simulink model "TST_EnvT_VD"  (R2016b)
settings: Solver=FixedStepDiscrete  StartTime=0.0  StopTime=simTime  FixedStep=sampleTime  RelTol=1e-3
values from neighbouring files (symbols this model uses):
  testCase = 1    [initTST_EnvT_VD_001.m]    (also in initTST_EnvT_VD_002.m = 2; initTST_EnvT_VD_003.m = 3; initTST_EnvT_VD_004.m = 4)
libraries: simulink x9, UnitTest_Lib x4
settings Model: Creator=liangyunbo  LastModifiedBy=liangyunbo
settings DebuggingCC: SignalRangeChecking=error

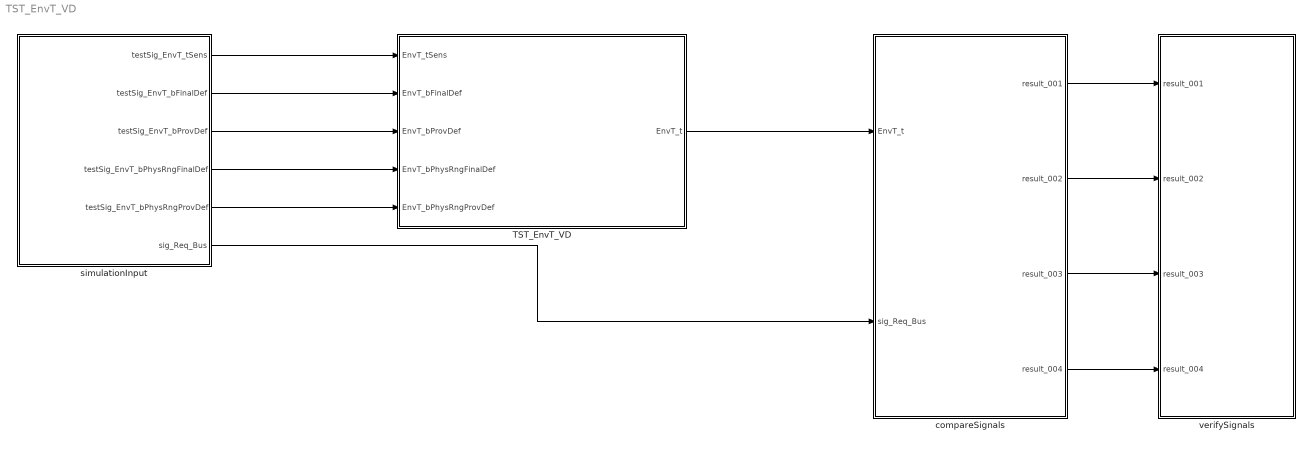
== system TST_EnvT_VD ==
  TST_EnvT_VD : Subsystem
  compareSignals : Subsystem
  simulationInput : Subsystem
  verifySignals : Subsystem
  wires:
  simulationInput/1(testSig_EnvT_tSens) -> TST_EnvT_VD/1(EnvT_tSens)
  simulationInput/2(testSig_EnvT_bFinalDef) -> TST_EnvT_VD/2(EnvT_bFinalDef)
  simulationInput/3(testSig_EnvT_bProvDef) -> TST_EnvT_VD/3(EnvT_bProvDef)
  simulationInput/4(testSig_EnvT_bPhysRngFinalDef) -> TST_EnvT_VD/4(EnvT_bPhysRngFinalDef)
  simulationInput/5(testSig_EnvT_bPhysRngProvDef) -> TST_EnvT_VD/5(EnvT_bPhysRngProvDef)
  TST_EnvT_VD/1(EnvT_t) -> compareSignals/1(EnvT_t)
  simulationInput/6(sig_Req_Bus) -> compareSignals/2(sig_Req_Bus)
  compareSignals/1(result_001) -> verifySignals/1(result_001)
  compareSignals/2(result_002) -> verifySignals/2(result_002)
  compareSignals/3(result_003) -> verifySignals/3(result_003)
  compareSignals/4(result_004) -> verifySignals/4(result_004)

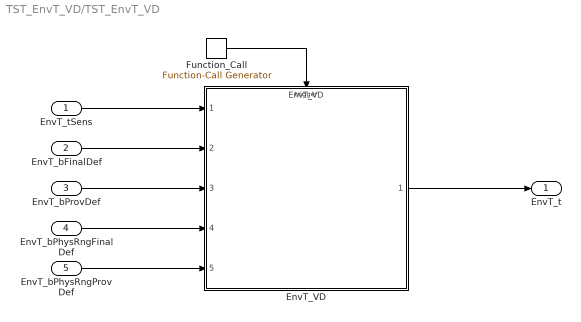
== system TST_EnvT_VD/TST_EnvT_VD ==
  EnvT_tSens : Inport
  EnvT_bFinalDef : Inport  Port=2
  EnvT_bProvDef : Inport  Port=3
  EnvT_bPhysRngFinalDef : Inport  Port=4
  EnvT_bPhysRngProvDef : Inport  Port=5
  EnvT_VD : ModelReference  ModelNameDialog=EnvT_VD  SimulationMode=Normal  ModelReferenceVersion=1.9  TriggerPortName=function  TriggerPortTriggerType=function-call  TriggerPortStatesWhenEnabling=held
  Function_Call : simulink/Ports & Subsystems/Function-Call Generator  sample_time=sampleTime  numberOfIterations=1
  EnvT_t : Outport
  wires:
  Function_Call/1 -> EnvT_VD/Trigger
  EnvT_tSens/1 -> EnvT_VD/1
  EnvT_bFinalDef/1 -> EnvT_VD/2
  EnvT_bProvDef/1 -> EnvT_VD/3
  EnvT_bPhysRngFinalDef/1 -> EnvT_VD/4
  EnvT_bPhysRngProvDef/1 -> EnvT_VD/5
  EnvT_VD/1 -> EnvT_t/1

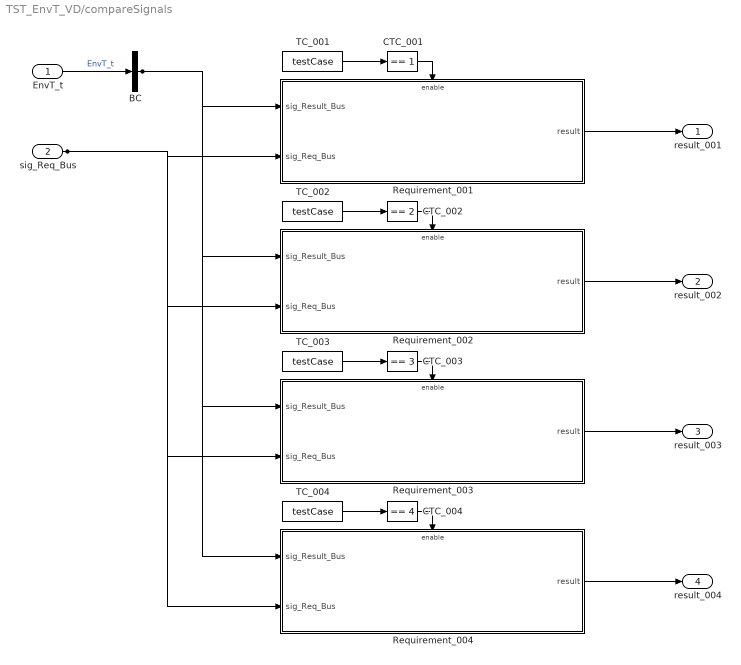
== system TST_EnvT_VD/compareSignals ==
  EnvT_t : Inport
  sig_Req_Bus : Inport  Port=2
  BC : BusCreator  Inputs=1
  CTC_001 : simulink/Logic and Bit Operations/Compare To Constant  relop===  const=1  OutDataTypeStr=boolean
  CTC_002 : simulink/Logic and Bit Operations/Compare To Constant  relop===  const=2  OutDataTypeStr=boolean
  CTC_003 : simulink/Logic and Bit Operations/Compare To Constant  relop===  const=3  OutDataTypeStr=boolean
  CTC_004 : simulink/Logic and Bit Operations/Compare To Constant  relop===  const=4  OutDataTypeStr=boolean
  Requirement_001 : Subsystem
  Requirement_002 : Subsystem
  Requirement_003 : Subsystem
  Requirement_004 : Subsystem
  TC_001 : Constant  Value=testCase
  TC_002 : Constant  Value=testCase
  TC_003 : Constant  Value=testCase
  TC_004 : Constant  Value=testCase
  result_001 : Outport
  result_002 : Outport  Port=2
  result_003 : Outport  Port=3
  result_004 : Outport  Port=4
  wires:
  EnvT_t/1 -> BC/1  "EnvT_t"
  TC_001/1 -> CTC_001/1
  CTC_001/1 -> Requirement_001/Enable
  sig_Req_Bus/1 -> Requirement_001/2(sig_Req_Bus), Requirement_002/2(sig_Req_Bus), Requirement_003/2(sig_Req_Bus), Requirement_004/2(sig_Req_Bus)
  BC/1 -> Requirement_001/1(sig_Result_Bus), Requirement_002/1(sig_Result_Bus), Requirement_003/1(sig_Result_Bus), Requirement_004/1(sig_Result_Bus)
  Requirement_001/1(result) -> result_001/1
  TC_002/1 -> CTC_002/1
  CTC_002/1 -> Requirement_002/Enable
  Requirement_002/1(result) -> result_002/1
  TC_003/1 -> CTC_003/1
  CTC_003/1 -> Requirement_003/Enable
  Requirement_003/1(result) -> result_003/1
  TC_004/1 -> CTC_004/1
  CTC_004/1 -> Requirement_004/Enable
  Requirement_004/1(result) -> result_004/1

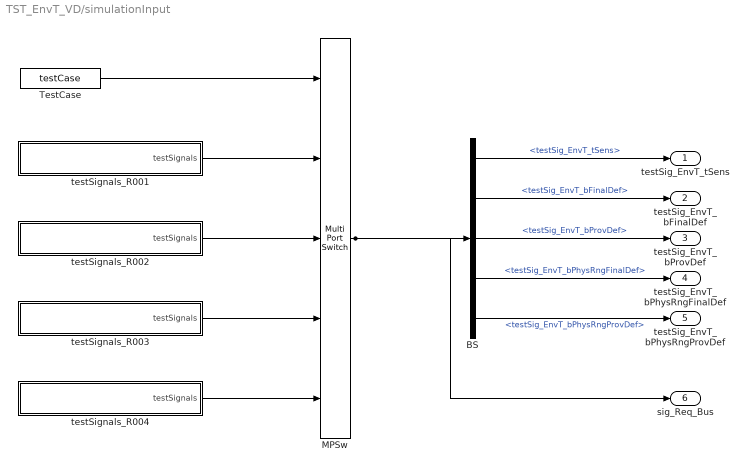
== system TST_EnvT_VD/simulationInput ==
  BS : BusSelector  OutputSignals=testSig_EnvT_tSens,testSig_EnvT_bFinalDef,testSig_EnvT_bProvDef,testSig_EnvT_bPhysRngFinalDef,testSig_EnvT_bPhysRngProvDef
  MPSw : MultiPortSwitch  Inputs=4  SaturateOnIntegerOverflow=on  InputSameDT=on
  TestCase : Constant  Value=testCase
  testSignals_R001 : Subsystem
  testSignals_R002 : Subsystem
  testSignals_R003 : Subsystem
  testSignals_R004 : Subsystem
  testSig_EnvT_tSens : Outport
  testSig_EnvT_bFinalDef : Outport  Port=2
  testSig_EnvT_bProvDef : Outport  Port=3
  testSig_EnvT_bPhysRngFinalDef : Outport  Port=4
  testSig_EnvT_bPhysRngProvDef : Outport  Port=5
  sig_Req_Bus : Outport  Port=6
  wires:
  BS/1 -> testSig_EnvT_tSens/1  "<testSig_EnvT_tSens>"
  BS/2 -> testSig_EnvT_bFinalDef/1  "<testSig_EnvT_bFinalDef>"
  BS/3 -> testSig_EnvT_bProvDef/1  "<testSig_EnvT_bProvDef>"
  BS/4 -> testSig_EnvT_bPhysRngFinalDef/1  "<testSig_EnvT_bPhysRngFinalDef>"
  BS/5 -> testSig_EnvT_bPhysRngProvDef/1  "<testSig_EnvT_bPhysRngProvDef>"
  MPSw/1 -> BS/1, sig_Req_Bus/1
  TestCase/1 -> MPSw/1
  testSignals_R001/1(testSignals) -> MPSw/2
  testSignals_R002/1(testSignals) -> MPSw/3
  testSignals_R003/1(testSignals) -> MPSw/4
  testSignals_R004/1(testSignals) -> MPSw/5

== system TST_EnvT_VD/verifySignals ==
  result_001 : Inport
  result_002 : Inport  Port=2
  result_003 : Inport  Port=3
  result_004 : Inport  Port=4
  Assertion_001 : Assertion  Enabled=off
  Assertion_002 : Assertion  Enabled=off
  Assertion_003 : Assertion  Enabled=off
  Assertion_004 : Assertion  Enabled=off
  wires:
  result_001/1 -> Assertion_001/1
  result_002/1 -> Assertion_002/1
  result_003/1 -> Assertion_003/1
  result_004/1 -> Assertion_004/1

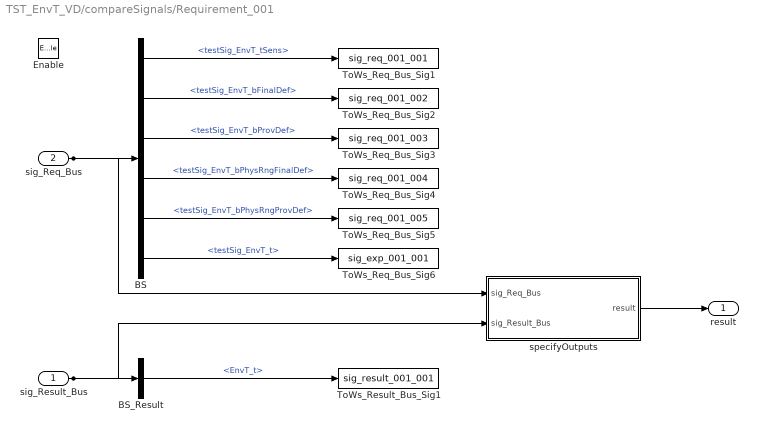
== system TST_EnvT_VD/compareSignals/Requirement_001 ==
  sig_Result_Bus : Inport
  sig_Req_Bus : Inport  Port=2
  Enable : EnablePort
  BS : BusSelector  OutputSignals=testSig_EnvT_tSens,testSig_EnvT_bFinalDef,testSig_EnvT_bProvDef,testSig_EnvT_bPhysRngFinalDef,testSig_EnvT_bPhysRngProvDef,testSig_EnvT_t
  BS_Result : BusSelector  OutputSignals=EnvT_t
  ToWs_Req_Bus_Sig1 : ToWorkspace  VariableName=sig_req_001_001  SaveFormat=Structure With Time
  ToWs_Req_Bus_Sig2 : ToWorkspace  VariableName=sig_req_001_002  SaveFormat=Structure With Time
  ToWs_Req_Bus_Sig3 : ToWorkspace  VariableName=sig_req_001_003  SaveFormat=Structure With Time
  ToWs_Req_Bus_Sig4 : ToWorkspace  VariableName=sig_req_001_004  SaveFormat=Structure With Time
  ToWs_Req_Bus_Sig5 : ToWorkspace  VariableName=sig_req_001_005  SaveFormat=Structure With Time
  ToWs_Req_Bus_Sig6 : ToWorkspace  VariableName=sig_exp_001_001  SaveFormat=Structure With Time
  ToWs_Result_Bus_Sig1 : ToWorkspace  VariableName=sig_result_001_001  SaveFormat=Structure With Time
  specifyOutputs : Subsystem
  result : Outport
  wires:
  sig_Req_Bus/1 -> BS/1, specifyOutputs/1(sig_Req_Bus)
  BS/1 -> ToWs_Req_Bus_Sig1/1  "<testSig_EnvT_tSens>"
  BS/2 -> ToWs_Req_Bus_Sig2/1  "<testSig_EnvT_bFinalDef>"
  BS/3 -> ToWs_Req_Bus_Sig3/1  "<testSig_EnvT_bProvDef>"
  BS/4 -> ToWs_Req_Bus_Sig4/1  "<testSig_EnvT_bPhysRngFinalDef>"
  BS/5 -> ToWs_Req_Bus_Sig5/1  "<testSig_EnvT_bPhysRngProvDef>"
  BS/6 -> ToWs_Req_Bus_Sig6/1  "<testSig_EnvT_t>"
  sig_Result_Bus/1 -> BS_Result/1, specifyOutputs/2(sig_Result_Bus)
  BS_Result/1 -> ToWs_Result_Bus_Sig1/1  "<EnvT_t>"
  specifyOutputs/1(result) -> result/1

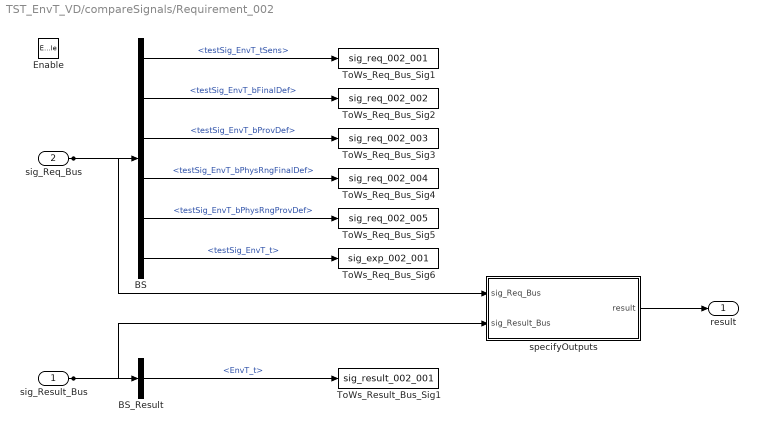
== system TST_EnvT_VD/compareSignals/Requirement_002 ==
  sig_Result_Bus : Inport
  sig_Req_Bus : Inport  Port=2
  Enable : EnablePort
  BS : BusSelector  OutputSignals=testSig_EnvT_tSens,testSig_EnvT_bFinalDef,testSig_EnvT_bProvDef,testSig_EnvT_bPhysRngFinalDef,testSig_EnvT_bPhysRngProvDef,testSig_EnvT_t
  BS_Result : BusSelector  OutputSignals=EnvT_t
  ToWs_Req_Bus_Sig1 : ToWorkspace  VariableName=sig_req_002_001  SaveFormat=Structure With Time
  ToWs_Req_Bus_Sig2 : ToWorkspace  VariableName=sig_req_002_002  SaveFormat=Structure With Time
  ToWs_Req_Bus_Sig3 : ToWorkspace  VariableName=sig_req_002_003  SaveFormat=Structure With Time
  ToWs_Req_Bus_Sig4 : ToWorkspace  VariableName=sig_req_002_004  SaveFormat=Structure With Time
  ToWs_Req_Bus_Sig5 : ToWorkspace  VariableName=sig_req_002_005  SaveFormat=Structure With Time
  ToWs_Req_Bus_Sig6 : ToWorkspace  VariableName=sig_exp_002_001  SaveFormat=Structure With Time
  ToWs_Result_Bus_Sig1 : ToWorkspace  VariableName=sig_result_002_001  SaveFormat=Structure With Time
  specifyOutputs : Subsystem
  result : Outport
  wires:
  sig_Req_Bus/1 -> BS/1, specifyOutputs/1(sig_Req_Bus)
  BS/1 -> ToWs_Req_Bus_Sig1/1  "<testSig_EnvT_tSens>"
  BS/2 -> ToWs_Req_Bus_Sig2/1  "<testSig_EnvT_bFinalDef>"
  BS/3 -> ToWs_Req_Bus_Sig3/1  "<testSig_EnvT_bProvDef>"
  BS/4 -> ToWs_Req_Bus_Sig4/1  "<testSig_EnvT_bPhysRngFinalDef>"
  BS/5 -> ToWs_Req_Bus_Sig5/1  "<testSig_EnvT_bPhysRngProvDef>"
  BS/6 -> ToWs_Req_Bus_Sig6/1  "<testSig_EnvT_t>"
  sig_Result_Bus/1 -> BS_Result/1, specifyOutputs/2(sig_Result_Bus)
  BS_Result/1 -> ToWs_Result_Bus_Sig1/1  "<EnvT_t>"
  specifyOutputs/1(result) -> result/1

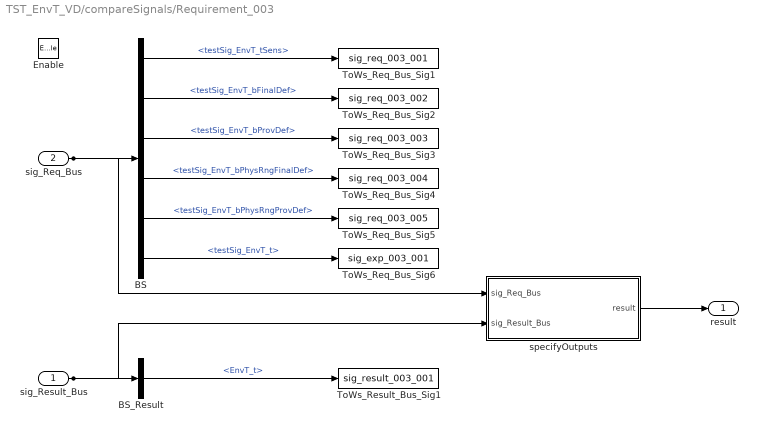
== system TST_EnvT_VD/compareSignals/Requirement_003 ==
  sig_Result_Bus : Inport
  sig_Req_Bus : Inport  Port=2
  Enable : EnablePort
  BS : BusSelector  OutputSignals=testSig_EnvT_tSens,testSig_EnvT_bFinalDef,testSig_EnvT_bProvDef,testSig_EnvT_bPhysRngFinalDef,testSig_EnvT_bPhysRngProvDef,testSig_EnvT_t
  BS_Result : BusSelector  OutputSignals=EnvT_t
  ToWs_Req_Bus_Sig1 : ToWorkspace  VariableName=sig_req_003_001  SaveFormat=Structure With Time
  ToWs_Req_Bus_Sig2 : ToWorkspace  VariableName=sig_req_003_002  SaveFormat=Structure With Time
  ToWs_Req_Bus_Sig3 : ToWorkspace  VariableName=sig_req_003_003  SaveFormat=Structure With Time
  ToWs_Req_Bus_Sig4 : ToWorkspace  VariableName=sig_req_003_004  SaveFormat=Structure With Time
  ToWs_Req_Bus_Sig5 : ToWorkspace  VariableName=sig_req_003_005  SaveFormat=Structure With Time
  ToWs_Req_Bus_Sig6 : ToWorkspace  VariableName=sig_exp_003_001  SaveFormat=Structure With Time
  ToWs_Result_Bus_Sig1 : ToWorkspace  VariableName=sig_result_003_001  SaveFormat=Structure With Time
  specifyOutputs : Subsystem
  result : Outport
  wires:
  sig_Req_Bus/1 -> BS/1, specifyOutputs/1(sig_Req_Bus)
  BS/1 -> ToWs_Req_Bus_Sig1/1  "<testSig_EnvT_tSens>"
  BS/2 -> ToWs_Req_Bus_Sig2/1  "<testSig_EnvT_bFinalDef>"
  BS/3 -> ToWs_Req_Bus_Sig3/1  "<testSig_EnvT_bProvDef>"
  BS/4 -> ToWs_Req_Bus_Sig4/1  "<testSig_EnvT_bPhysRngFinalDef>"
  BS/5 -> ToWs_Req_Bus_Sig5/1  "<testSig_EnvT_bPhysRngProvDef>"
  BS/6 -> ToWs_Req_Bus_Sig6/1  "<testSig_EnvT_t>"
  sig_Result_Bus/1 -> BS_Result/1, specifyOutputs/2(sig_Result_Bus)
  BS_Result/1 -> ToWs_Result_Bus_Sig1/1  "<EnvT_t>"
  specifyOutputs/1(result) -> result/1

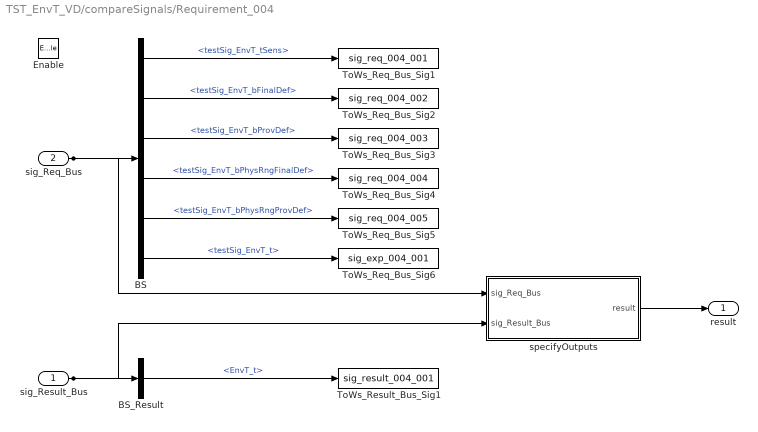
== system TST_EnvT_VD/compareSignals/Requirement_004 ==
  sig_Result_Bus : Inport
  sig_Req_Bus : Inport  Port=2
  Enable : EnablePort
  BS : BusSelector  OutputSignals=testSig_EnvT_tSens,testSig_EnvT_bFinalDef,testSig_EnvT_bProvDef,testSig_EnvT_bPhysRngFinalDef,testSig_EnvT_bPhysRngProvDef,testSig_EnvT_t
  BS_Result : BusSelector  OutputSignals=EnvT_t
  ToWs_Req_Bus_Sig1 : ToWorkspace  VariableName=sig_req_004_001  SaveFormat=Structure With Time
  ToWs_Req_Bus_Sig2 : ToWorkspace  VariableName=sig_req_004_002  SaveFormat=Structure With Time
  ToWs_Req_Bus_Sig3 : ToWorkspace  VariableName=sig_req_004_003  SaveFormat=Structure With Time
  ToWs_Req_Bus_Sig4 : ToWorkspace  VariableName=sig_req_004_004  SaveFormat=Structure With Time
  ToWs_Req_Bus_Sig5 : ToWorkspace  VariableName=sig_req_004_005  SaveFormat=Structure With Time
  ToWs_Req_Bus_Sig6 : ToWorkspace  VariableName=sig_exp_004_001  SaveFormat=Structure With Time
  ToWs_Result_Bus_Sig1 : ToWorkspace  VariableName=sig_result_004_001  SaveFormat=Structure With Time
  specifyOutputs : Subsystem
  result : Outport
  wires:
  sig_Req_Bus/1 -> BS/1, specifyOutputs/1(sig_Req_Bus)
  BS/1 -> ToWs_Req_Bus_Sig1/1  "<testSig_EnvT_tSens>"
  BS/2 -> ToWs_Req_Bus_Sig2/1  "<testSig_EnvT_bFinalDef>"
  BS/3 -> ToWs_Req_Bus_Sig3/1  "<testSig_EnvT_bProvDef>"
  BS/4 -> ToWs_Req_Bus_Sig4/1  "<testSig_EnvT_bPhysRngFinalDef>"
  BS/5 -> ToWs_Req_Bus_Sig5/1  "<testSig_EnvT_bPhysRngProvDef>"
  BS/6 -> ToWs_Req_Bus_Sig6/1  "<testSig_EnvT_t>"
  sig_Result_Bus/1 -> BS_Result/1, specifyOutputs/2(sig_Result_Bus)
  BS_Result/1 -> ToWs_Result_Bus_Sig1/1  "<EnvT_t>"
  specifyOutputs/1(result) -> result/1

== system TST_EnvT_VD/simulationInput/testSignals_R001 ==
  BC : BusCreator  Inputs=6
  spec_EnvT_bFinalDef : FromWorkspace  VariableName=testSig_EnvT_bFinalDef  Interpolate=off  OutputAfterFinalValue=Holding final value
  spec_EnvT_bPhysRngFinalDef : FromWorkspace  VariableName=testSig_EnvT_bPhysRngFinalDef  Interpolate=off  OutputAfterFinalValue=Holding final value
  spec_EnvT_bPhysRngProvDef : FromWorkspace  VariableName=testSig_EnvT_bPhysRngProvDef  Interpolate=off  OutputAfterFinalValue=Holding final value
  spec_EnvT_bProvDef : FromWorkspace  VariableName=testSig_EnvT_bProvDef  Interpolate=off  OutputAfterFinalValue=Holding final value
  spec_EnvT_t : FromWorkspace  VariableName=testSig_EnvT_t  Interpolate=off  OutputAfterFinalValue=Holding final value
  spec_EnvT_tSens : FromWorkspace  VariableName=testSig_EnvT_tSens  Interpolate=off  OutputAfterFinalValue=Holding final value
  testSignals : Outport
  wires:
  BC/1 -> testSignals/1
  spec_EnvT_tSens/1 -> BC/1  "testSig_EnvT_tSens"
  spec_EnvT_bFinalDef/1 -> BC/2  "testSig_EnvT_bFinalDef"
  spec_EnvT_bProvDef/1 -> BC/3  "testSig_EnvT_bProvDef"
  spec_EnvT_bPhysRngFinalDef/1 -> BC/4  "testSig_EnvT_bPhysRngFinalDef"
  spec_EnvT_bPhysRngProvDef/1 -> BC/5  "testSig_EnvT_bPhysRngProvDef"
  spec_EnvT_t/1 -> BC/6  "testSig_EnvT_t"

== system TST_EnvT_VD/simulationInput/testSignals_R002 ==
  BC : BusCreator  Inputs=6
  spec_EnvT_bFinalDef : FromWorkspace  VariableName=testSig_EnvT_bFinalDef  Interpolate=off  OutputAfterFinalValue=Holding final value
  spec_EnvT_bPhysRngFinalDef : FromWorkspace  VariableName=testSig_EnvT_bPhysRngFinalDef  Interpolate=off  OutputAfterFinalValue=Holding final value
  spec_EnvT_bPhysRngProvDef : FromWorkspace  VariableName=testSig_EnvT_bPhysRngProvDef  Interpolate=off  OutputAfterFinalValue=Holding final value
  spec_EnvT_bProvDef : FromWorkspace  VariableName=testSig_EnvT_bProvDef  Interpolate=off  OutputAfterFinalValue=Holding final value
  spec_EnvT_t : FromWorkspace  VariableName=testSig_EnvT_t  Interpolate=off  OutputAfterFinalValue=Holding final value
  spec_EnvT_tSens : FromWorkspace  VariableName=testSig_EnvT_tSens  Interpolate=off  OutputAfterFinalValue=Holding final value
  testSignals : Outport
  wires:
  BC/1 -> testSignals/1
  spec_EnvT_tSens/1 -> BC/1  "testSig_EnvT_tSens"
  spec_EnvT_bFinalDef/1 -> BC/2  "testSig_EnvT_bFinalDef"
  spec_EnvT_bProvDef/1 -> BC/3  "testSig_EnvT_bProvDef"
  spec_EnvT_bPhysRngFinalDef/1 -> BC/4  "testSig_EnvT_bPhysRngFinalDef"
  spec_EnvT_bPhysRngProvDef/1 -> BC/5  "testSig_EnvT_bPhysRngProvDef"
  spec_EnvT_t/1 -> BC/6  "testSig_EnvT_t"

== system TST_EnvT_VD/simulationInput/testSignals_R003 ==
  BC : BusCreator  Inputs=6
  spec_EnvT_bFinalDef : FromWorkspace  VariableName=testSig_EnvT_bFinalDef  Interpolate=off  OutputAfterFinalValue=Holding final value
  spec_EnvT_bPhysRngFinalDef : FromWorkspace  VariableName=testSig_EnvT_bPhysRngFinalDef  Interpolate=off  OutputAfterFinalValue=Holding final value
  spec_EnvT_bPhysRngProvDef : FromWorkspace  VariableName=testSig_EnvT_bPhysRngProvDef  Interpolate=off  OutputAfterFinalValue=Holding final value
  spec_EnvT_bProvDef : FromWorkspace  VariableName=testSig_EnvT_bProvDef  Interpolate=off  OutputAfterFinalValue=Holding final value
  spec_EnvT_t : FromWorkspace  VariableName=testSig_EnvT_t  Interpolate=off  OutputAfterFinalValue=Holding final value
  spec_EnvT_tSens : FromWorkspace  VariableName=testSig_EnvT_tSens  Interpolate=off  OutputAfterFinalValue=Holding final value
  testSignals : Outport
  wires:
  BC/1 -> testSignals/1
  spec_EnvT_tSens/1 -> BC/1  "testSig_EnvT_tSens"
  spec_EnvT_bFinalDef/1 -> BC/2  "testSig_EnvT_bFinalDef"
  spec_EnvT_bProvDef/1 -> BC/3  "testSig_EnvT_bProvDef"
  spec_EnvT_bPhysRngFinalDef/1 -> BC/4  "testSig_EnvT_bPhysRngFinalDef"
  spec_EnvT_bPhysRngProvDef/1 -> BC/5  "testSig_EnvT_bPhysRngProvDef"
  spec_EnvT_t/1 -> BC/6  "testSig_EnvT_t"

== system TST_EnvT_VD/simulationInput/testSignals_R004 ==
  BC : BusCreator  Inputs=6
  spec_EnvT_bFinalDef : FromWorkspace  VariableName=testSig_EnvT_bFinalDef  Interpolate=off  OutputAfterFinalValue=Holding final value
  spec_EnvT_bPhysRngFinalDef : FromWorkspace  VariableName=testSig_EnvT_bPhysRngFinalDef  Interpolate=off  OutputAfterFinalValue=Holding final value
  spec_EnvT_bPhysRngProvDef : FromWorkspace  VariableName=testSig_EnvT_bPhysRngProvDef  Interpolate=off  OutputAfterFinalValue=Holding final value
  spec_EnvT_bProvDef : FromWorkspace  VariableName=testSig_EnvT_bProvDef  Interpolate=off  OutputAfterFinalValue=Holding final value
  spec_EnvT_t : FromWorkspace  VariableName=testSig_EnvT_t  Interpolate=off  OutputAfterFinalValue=Holding final value
  spec_EnvT_tSens : FromWorkspace  VariableName=testSig_EnvT_tSens  Interpolate=off  OutputAfterFinalValue=Holding final value
  testSignals : Outport
  wires:
  BC/1 -> testSignals/1
  spec_EnvT_tSens/1 -> BC/1  "testSig_EnvT_tSens"
  spec_EnvT_bFinalDef/1 -> BC/2  "testSig_EnvT_bFinalDef"
  spec_EnvT_bProvDef/1 -> BC/3  "testSig_EnvT_bProvDef"
  spec_EnvT_bPhysRngFinalDef/1 -> BC/4  "testSig_EnvT_bPhysRngFinalDef"
  spec_EnvT_bPhysRngProvDef/1 -> BC/5  "testSig_EnvT_bPhysRngProvDef"
  spec_EnvT_t/1 -> BC/6  "testSig_EnvT_t"

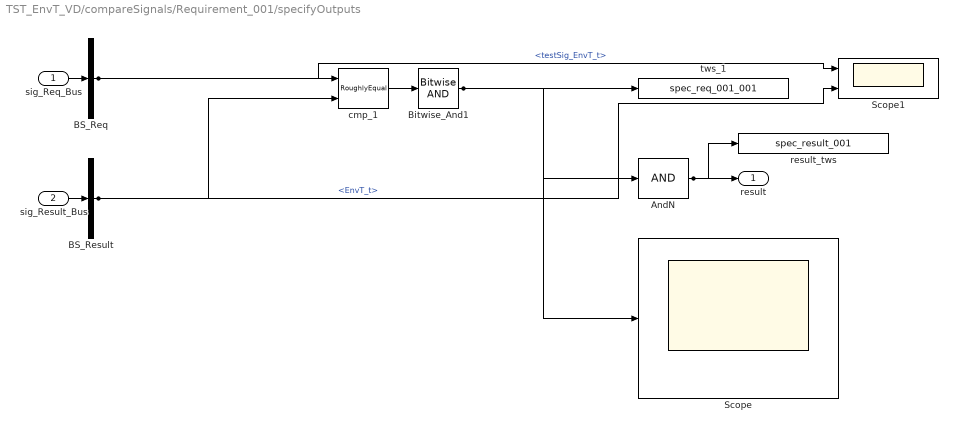
== system TST_EnvT_VD/compareSignals/Requirement_001/specifyOutputs ==
  sig_Req_Bus : Inport
  sig_Result_Bus : Inport  Port=2
  AndN : Logic  Inputs=1
  BS_Req : BusSelector  OutputSignals=testSig_EnvT_t
  BS_Result : BusSelector  OutputSignals=EnvT_t
  Bitwise_And1 : simulink/Logic and Bit Operations/Bitwise Operator  logicop=AND  UseBitMask=off  BitMask=bin2dec('11011001')  BitMaskRealWorld=Stored Integer
  Scope : Scope
  Scope1 : Scope  NumInputPorts=2
  cmp_1 : UnitTest_Lib/RoughlyEqual  slope=0.1
  result_tws : ToWorkspace  VariableName=spec_result_001
  tws_1 : ToWorkspace  VariableName=spec_req_001_001
  result : Outport
  wires:
  sig_Req_Bus/1 -> BS_Req/1
  sig_Result_Bus/1 -> BS_Result/1
  AndN/1 -> result/1, result_tws/1
  BS_Req/1 -> cmp_1/1, Scope1/1  "<testSig_EnvT_t>"
  BS_Result/1 -> cmp_1/2, Scope1/2  "<EnvT_t>"
  cmp_1/1 -> Bitwise_And1/1
  Bitwise_And1/1 -> tws_1/1, AndN/1, Scope/1

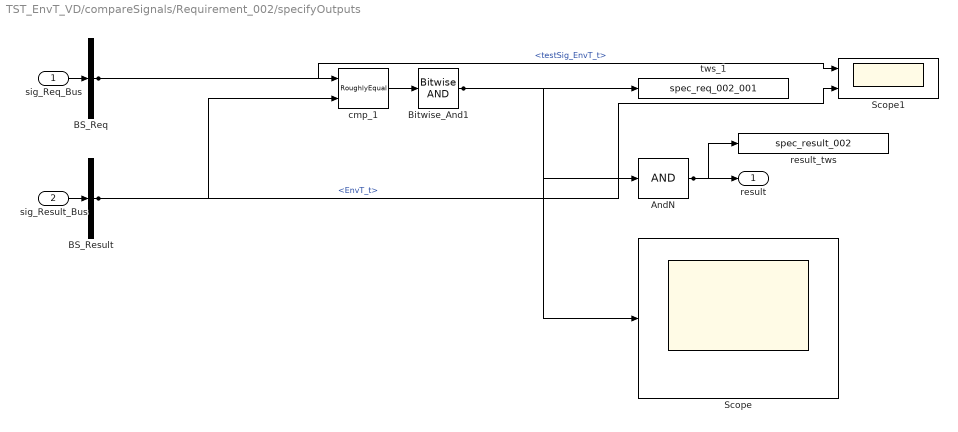
== system TST_EnvT_VD/compareSignals/Requirement_002/specifyOutputs ==
  sig_Req_Bus : Inport
  sig_Result_Bus : Inport  Port=2
  AndN : Logic  Inputs=1
  BS_Req : BusSelector  OutputSignals=testSig_EnvT_t
  BS_Result : BusSelector  OutputSignals=EnvT_t
  Bitwise_And1 : simulink/Logic and Bit Operations/Bitwise Operator  logicop=AND  UseBitMask=off  BitMask=bin2dec('11011001')  BitMaskRealWorld=Stored Integer
  Scope : Scope
  Scope1 : Scope  NumInputPorts=2
  cmp_1 : UnitTest_Lib/RoughlyEqual  slope=0.1
  result_tws : ToWorkspace  VariableName=spec_result_002
  tws_1 : ToWorkspace  VariableName=spec_req_002_001
  result : Outport
  wires:
  sig_Req_Bus/1 -> BS_Req/1
  sig_Result_Bus/1 -> BS_Result/1
  AndN/1 -> result/1, result_tws/1
  BS_Req/1 -> cmp_1/1, Scope1/1  "<testSig_EnvT_t>"
  BS_Result/1 -> cmp_1/2, Scope1/2  "<EnvT_t>"
  cmp_1/1 -> Bitwise_And1/1
  Bitwise_And1/1 -> tws_1/1, AndN/1, Scope/1

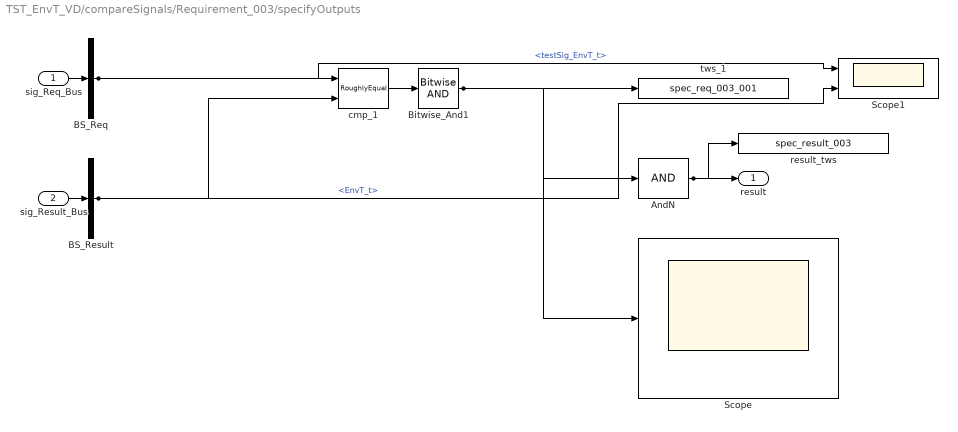
== system TST_EnvT_VD/compareSignals/Requirement_003/specifyOutputs ==
  sig_Req_Bus : Inport
  sig_Result_Bus : Inport  Port=2
  AndN : Logic  Inputs=1
  BS_Req : BusSelector  OutputSignals=testSig_EnvT_t
  BS_Result : BusSelector  OutputSignals=EnvT_t
  Bitwise_And1 : simulink/Logic and Bit Operations/Bitwise Operator  logicop=AND  UseBitMask=off  BitMask=bin2dec('11011001')  BitMaskRealWorld=Stored Integer
  Scope : Scope
  Scope1 : Scope  NumInputPorts=2
  cmp_1 : UnitTest_Lib/RoughlyEqual  slope=0.1
  result_tws : ToWorkspace  VariableName=spec_result_003
  tws_1 : ToWorkspace  VariableName=spec_req_003_001
  result : Outport
  wires:
  sig_Req_Bus/1 -> BS_Req/1
  sig_Result_Bus/1 -> BS_Result/1
  AndN/1 -> result/1, result_tws/1
  BS_Req/1 -> cmp_1/1, Scope1/1  "<testSig_EnvT_t>"
  BS_Result/1 -> cmp_1/2, Scope1/2  "<EnvT_t>"
  cmp_1/1 -> Bitwise_And1/1
  Bitwise_And1/1 -> tws_1/1, AndN/1, Scope/1

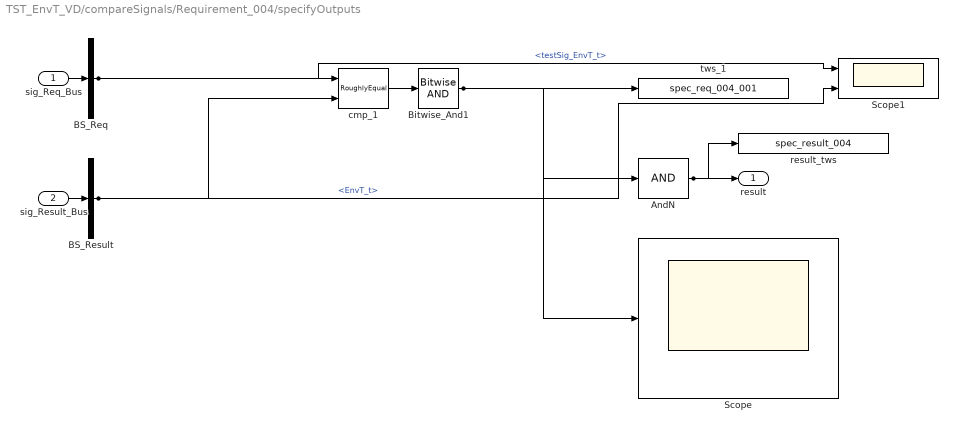
== system TST_EnvT_VD/compareSignals/Requirement_004/specifyOutputs ==
  sig_Req_Bus : Inport
  sig_Result_Bus : Inport  Port=2
  AndN : Logic  Inputs=1
  BS_Req : BusSelector  OutputSignals=testSig_EnvT_t
  BS_Result : BusSelector  OutputSignals=EnvT_t
  Bitwise_And1 : simulink/Logic and Bit Operations/Bitwise Operator  logicop=AND  UseBitMask=off  BitMask=bin2dec('11011001')  BitMaskRealWorld=Stored Integer
  Scope : Scope
  Scope1 : Scope  NumInputPorts=2
  cmp_1 : UnitTest_Lib/RoughlyEqual  slope=0.1
  result_tws : ToWorkspace  VariableName=spec_result_004
  tws_1 : ToWorkspace  VariableName=spec_req_004_001
  result : Outport
  wires:
  sig_Req_Bus/1 -> BS_Req/1
  sig_Result_Bus/1 -> BS_Result/1
  AndN/1 -> result/1, result_tws/1
  BS_Req/1 -> cmp_1/1, Scope1/1  "<testSig_EnvT_t>"
  BS_Result/1 -> cmp_1/2, Scope1/2  "<EnvT_t>"
  cmp_1/1 -> Bitwise_And1/1
  Bitwise_And1/1 -> tws_1/1, AndN/1, Scope/1
